simulink model "SquatTrotClimbRefined"  (R2025b)
settings: Solver=ode45  StartTime=0.0  StopTime=200  MaxStep=0.002  RelTol=0.01  AbsTol=0.01  EnableMultiTasking=on
undefined symbols (not defined in the file): a, b, c, waypoints, X, Y, Z
libraries: sm_lib x81, nesl_utility x67, hdlsllib x12, slpidlib x2, robotalgslib x1, sharedtransform x1
(part 6 of 6)

== matlab function SquatTrotClimbRefined/Rear_left_gait/MATLAB Function2 ==
  data: t input; leg_id input; q_hip output; mode_cmd input
function q_hip = hip_motion_all_legs(t, leg_id, mode_cmd)
    T_squat_start = 102;
    T_walk_start  = 130;
    
    % --- [NEW] Absolute time node for ending the walk ---
    T_walk_end    = 170;  % Start braking and retracting legs exactly at 170 seconds
    
    if (mode_cmd == 1) || (t < T_squat_start)
        q_hip = 0; return;
    end
    
    % Phase 1: Squat and stand (102s - 130s)
    if t < T_walk_start
        tau = t - T_squat_start;
        q_stand = 0; q_squat = deg2rad(35);
        T1=3; T2=15; T3=3;
        
        if tau < T1
            u = tau/T1; 
            q_hip = (1-u)*q_stand + u*q_squat;
        elseif tau < T1+T2
            q_hip = q_squat;
        elseif tau < T1+T2+T3
            u = (tau-(T1+T2))/T3; 
            q_hip = (1-u)*q_squat + u*q_stand;
        else
            q_hip = 0; 
        end
        return;
    end
    
    % Phase 2: Walking logic (130s+)
    % Relative time starting from 130s
    t_phase2 = t - T_walk_start;
    
    % ================= Tunables (Hip) =================
    ang_hip_crouch = deg2rad(30);    
    hip_swing_amp  = deg2rad(8);     
    
    ang_fwd  = ang_hip_crouch - hip_swing_amp;  
    ang_back = ang_hip_crouch + hip_swing_amp;  
    
    % ================= Timing =================
    T_crouch = 2.0;              
    T_hold   = 3.0;              
    T_ramp   = 2.0;              
    T_cycle  = 1.8;
    duty     = 0.50;             
    
    % --- [NEW] Braking and recovery time periods ---
    T_ramp_down = 2.0;    % 170s - 172s: Take 2 seconds to slowly reduce stride amplitude to 0
    T_recover   = 3.0;    % 172s - 175s: After legs stop, take 3 seconds to smoothly stand up straight (return to 0 degrees)
    
    % ================= Phase offsets =================
    phase_offset = [0.0, 0.5, 0.0, 0.5];
    phi = phase_offset(leg_id + 1);
    
    % ================= Smooth interpolators =================
    smooth = @(x) (1 - cos(x * pi)) / 2;
    
    % ==========================================================
    % Stage 1 & 2: Crouch & Hold (relative to 130s) -> (130s ~ 135s)
    % ==========================================================
    if t_phase2 < T_crouch + T_hold
        s = smooth(min(t_phase2 / T_crouch, 1.0));
        q_hip = s * ang_hip_crouch;
        return;
    end
    
    % ==========================================================
    % Stage 3: Trot & Stop (All motions after 135s)
    % ==========================================================
    t_trot = t_phase2 - T_crouch - T_hold;
    phase = mod(t_trot / T_cycle + phi, 1.0);
    
    % --- 1. Calculate theoretical pure gait trajectory (keep your already tuned normal logic) ---
    if phase < duty
        % ===== STANCE =====
        s = smooth(phase / duty);
        hip_walk  = ang_fwd + s * (ang_back - ang_fwd); 
    else
        % ===== SWING =====
        s = (phase - duty) / (1.0 - duty);
        hip_walk  = ang_back + smooth(s) * (ang_fwd - ang_back);
    end
    
    % Extract the pure stepping swing amount
    swing_offset = hip_walk - ang_hip_crouch;
    
    % --- 2. Calculate stride amplitude envelope (controls how large the step is) ---
    if t < T_walk_end
        % 135s - 170s: Start and maintain full speed
        amp_walk = smooth(min(t_trot / T_ramp, 1.0));
    elseif t < T_walk_end + T_ramp_down
        % 170s - 172s: Stride amplitude gradually decreases until stopping in place
        tau_stop = t - T_walk_end;
        amp_walk = smooth(max(1.0 - (tau_stop / T_ramp_down), 0.0));
    else
        % After 172s: Legs completely stop stepping
        amp_walk = 0.0;
    end
    
    % --- 3. Calculate base crouch angle (controls body height) ---
    if t < T_walk_end + T_ramp_down
        % Before 172s: Maintain 30 degree crouch baseline
        base_hip = ang_hip_crouch;
    elseif t < T_walk_end + T_ramp_down + T_recover
        % 172s - 175s: Smoothly stand up from 30 degree crouch back to 0 degrees
        tau_rec = t - (T_walk_end + T_ramp_down);
        s_rec = smooth(min(tau_rec / T_recover, 1.0));
        base_hip = (1.0 - s_rec) * ang_hip_crouch;
    else
        % After 175s: Completely stand straight, lock at 0 degrees, and enter wheeled driving mode
        base_hip = 0.0;
    end
    
    % --- 4. Final output = Base posture + (Stride proportion * Swing amount) ---
    q_hip = base_hip + amp_walk * swing_offset;
end

== matlab function SquatTrotClimbRefined/Rear_left_gait/MATLAB Function4 ==
  data: t input; leg_id input; q_knee output; mode_cmd input
function q_knee = knee_motion_all_legs(t, leg_id, mode_cmd)
    % --- Time Node Definitions ---
    T_squat_start = 102;
    T_walk_start  = 130; 
    
    % --- [NEW] Absolute time node for ending the walk ---
    T_walk_end    = 170;  
    
    % Phase 0: Standby
    if (mode_cmd == 1) || (t < T_squat_start)
        q_knee = 0; return;
    end
    
    % Phase 1: Squat and stand (102-130s)
    if t < T_walk_start
        tau = t - T_squat_start;
        q_stand = 0; q_squat = -deg2rad(70);
        T1=3; T2=15; T3=3;
        
        if tau < T1
            u = tau/T1; 
            q_knee = (1-u)*q_stand + u*q_squat;
        elseif tau < T1+T2
            q_knee = q_squat;
        elseif tau < T1+T2+T3
            u = (tau-(T1+T2))/T3; 
            q_knee = (1-u)*q_squat + u*q_stand;
        else
            q_knee = 0; 
        end
        return;
    end
    
    % Phase 2: Walking logic (130s+)
    % Relative time starting from 130s
    t_phase2 = t - T_walk_start;
    
    % ================= Tunables (Knee) =================
    ang_crouch = deg2rad(-40);   % Base walking crouch angle
    ang_lift   = deg2rad(-8);    % Leg lift amplitude during swing
    ang_comp   = deg2rad(-3);    % Compression amplitude during stance
    
    % ================= Timing =================
    T_crouch = 2.0;              
    T_hold   = 3.0;              
    T_ramp   = 2.0;              
    T_cycle  = 1.8;
    duty     = 0.50;             
    
    % --- [NEW] Braking and recovery time periods ---
    T_ramp_down = 2.0;    % 170s - 172s: Take 2 seconds to slowly reduce the step amplitude to 0
    T_recover   = 3.0;    % 172s - 175s: After the legs stop, take 3 seconds to smoothly stand up straight (return to 0 degrees)
    
    % ================= Phase offsets =================
    phase_offset = [0.0, 0.5, 0.0, 0.5];
    phi = phase_offset(leg_id + 1);
    
    % ================= Smooth interpolators =================
    smooth = @(x) (1 - cos(x * pi)) / 2;
    bump   = @(x) (1 - cos(2 * x * pi)) / 2;
    
    % ==========================================================
    % Stage 1 & 2: Crouch & Hold (relative to 130s) -> (130s ~ 135s)
    % ==========================================================
    if t_phase2 < T_crouch + T_hold
        s = smooth(min(t_phase2 / T_crouch, 1.0));
        q_knee = s * ang_crouch;
        return;
    end
    
    % ==========================================================
    % Stage 3: Trot & Stop (All motions after 135s)
    % ==========================================================
    t_trot = t_phase2 - T_crouch - T_hold;
    phase = mod(t_trot / T_cycle + phi, 1.0);
    
    % --- 1. Calculate theoretical pure gait trajectory (keep calculating normally to prevent phase disruption from sudden cutoff) ---
    if phase < duty
        % ===== STANCE: foot on ground =====
        knee_walk = ang_crouch + sin((phase / duty) * pi) * ang_comp;
    else
        % ===== SWING: foot in air =====
        s = (phase - duty) / (1.0 - duty);
        knee_walk = ang_crouch + bump(s) * ang_lift;
    end
    
    % Extract the pure stepping flexion/extension amount
    swing_offset = knee_walk - ang_crouch;
    
    % --- 2. Calculate stride amplitude envelope (controls how large the step is) ---
    if t < T_walk_end
        % 135s - 170s: Start and maintain full-amplitude stepping
        amp_walk = smooth(min(t_trot / T_ramp, 1.0));
    elseif t < T_walk_end + T_ramp_down
        % 170s - 172s: Stride amplitude gradually decreases until stopping in place
        tau_stop = t - T_walk_end;
        amp_walk = smooth(max(1.0 - (tau_stop / T_ramp_down), 0.0));
    else
        % After 172s: Legs completely stop stepping
        amp_walk = 0.0;
    end
    
    % --- 3. Calculate base crouch angle (controls body height) ---
    if t < T_walk_end + T_ramp_down
        % Before 172s: Maintain -40 degree crouch baseline
        base_knee = ang_crouch;
    elseif t < T_walk_end + T_ramp_down + T_recover
        % 172s - 175s: Smoothly stand up from -40 degrees back to 0 degrees
        tau_rec = t - (T_walk_end + T_ramp_down);
        s_rec = smooth(min(tau_rec / T_recover, 1.0));
        base_knee = (1.0 - s_rec) * ang_crouch;
    else
        % After 175s: Completely stand straight, lock at 0 degrees, and enter wheeled driving mode
        base_knee = 0.0;
    end
    
    % --- 4. Final synthesis ---
    % Final output = Base knee angle + (Stride proportion * Additional flexion/extension amount)
    q_knee = base_knee + amp_walk * swing_offset;
end

== matlab function SquatTrotClimbRefined/RL/MATLAB Function4 ==
  data: t input; w output
function w = wheel_speed(t)
% WHEEL_SPEED_CONTROLLER 
% This function manages the angular velocity for the rear wheels.
% Sequence: High-speed drive -> Stop -> WALKING GAIT (130s-175s) -> Low-speed drive -> Stop 10s -> Drive.

% ==========================================
% 1. Parameter Definitions (Phase 1 to 5: Initial Drive)
% ==========================================
T_start    = 105;   % Time to begin initial movement (s)
T_accel    = 2;     % Duration of linear acceleration (s)
V_max      = 100;   % Primary target velocity
V_low      = 15;    % Secondary target velocity (used in intermediate phases)
T_dec_init = 125;   % Time to start the first deceleration (s)
T_braking  = 3;     % Duration of the braking phase (s)

% ==========================================
% 2. Parameter Definitions (Phase 6+: Resume Drive after 175s)
% ==========================================
T_resume   = 175;   % Time to resume wheeled mode (Walking gait ends)
T_accel2   = 2;     % Duration to accelerate to V_low
T_hold2    = 8;     % Duration to hold V_low before the second stop
T_brake2   = 3;     % Duration of the second braking phase
T_pause2   = 2;    % Pause duration (Stop for 10s)
T_accel3   = 2;     % Final acceleration duration to V_low

% --- Pre-calculate Time Nodes for clean logic ---
T1_end_dec   = T_dec_init + T_braking; % 128s: First stop completely

T2_end_accel = T_resume + T_accel2;    % 177s: Reached 20 rad/s
T2_start_dec = T2_end_accel + T_hold2; % 185s: Start 2nd braking
T2_end_dec   = T2_start_dec + T_brake2;% 188s: Completely stopped again
T2_end_pause = T2_end_dec + T_pause2;  % 198s: 10s pause ends
T3_end_accel = T2_end_pause + T_accel3;% 200s: Final acceleration ends

% ==========================================
% 3. Logic Control and Phase Switching
% ==========================================

% --- PHASE 1: IDLE / PRE-START ---
if t < T_start
    w = 0;

% --- PHASE 2: INITIAL ACCELERATION (0 to V_max) ---
elseif t < T_start + T_accel
    u = (t - T_start) / T_accel; 
    w = u * V_max;

% --- PHASE 3: CONSTANT HIGH-SPEED CRUISE ---
elseif t < T_dec_init
    w = V_max;

% --- PHASE 4: CONTROLLED DECELERATION (V_max to 0) ---
elseif t < T1_end_dec
    u = (t - T_dec_init) / T_braking; 
    w = V_max * (1 - u);

% =========================================================
% --- PHASE 5: WALKING GAIT LOCK (128s to 175s) ---
% The robot stands still from 128s-130s, then walks from 130s-175s.
% Wheels MUST strictly remain at 0 rad/s here.
% =========================================================
elseif t < T_resume
    w = 0;

% =========================================================
% --- PHASE 6+: RESUME WHEELED MODE (175s onwards) ---
% =========================================================

% --- PHASE 6: FIRST RE-ACCELERATION (0 to V_low) ---
elseif t < T2_end_accel
    u = (t - T_resume) / T_accel2;
    w = u * V_low;

% --- PHASE 7: HOLD V_low ---
elseif t < T2_start_dec
    w = V_low;

% --- PHASE 8: SECOND DECELERATION (V_low to 0) ---
elseif t < T2_end_dec
    u = (t - T2_start_dec) / T_brake2;
    w = V_low * (1 - u);

% --- PHASE 9: THE 10-SECOND PAUSE ---
elseif t < T2_end_pause
    w = 0;

% --- PHASE 10: FINAL ACCELERATION (0 to V_low) ---
elseif t < T3_end_accel
    u = (t - T2_end_pause) / T_accel3;
    w = u * V_low;

% --- PHASE 11: CRUISE INDEFINITELY ---
else
    w = V_low;
end

end

== matlab function SquatTrotClimbRefined/RR/MATLAB Function ==
  data: mode_cmd input; alpha input; tau output; q input; dq input; q_cmd input; is_locked output; q_ref output
function [tau, is_locked, q_ref] = LockJointPD(mode_cmd, alpha, q, dq, q_cmd)
%#codegen
% mode_cmd: 0=Walk(folloew q_cmd), 1=Wheel(lock the present angle )
% alpha   : [0,1] flatten faktor(TransferFcnoutput)，0=walk, 1=leg locked
% q,dq    : joint angle/angular velocity
% q_cmd   : walking/standing angle(rad)

Kp = 1200.0;   % start value
Kd =   20.0;
tau_lim = 300.0;

m = uint8(mode_cmd ~= 0);     % uint8(0/1)
a = double(alpha);

persistent q_hold last_mode
if isempty(q_hold),    q_hold    = q;        end   % double
if isempty(last_mode), last_mode = uint8(0); end   % uint8

% step: 0->1 
if (last_mode == uint8(0)) && (m ~= uint8(0))
    q_hold = q;
end
last_mode = m;

% reference angle
q_ref  = a*q_hold + (1-a)*q_cmd;
dq_ref = 0.0;

% PD
tau = Kp*(q_ref - q) + Kd*(dq_ref - dq);

% 
tau = max(min(tau, tau_lim), -tau_lim);

% 
is_locked = (a > 0.5);     % 
end

== matlab function SquatTrotClimbRefined/FR/MATLAB Function ==
  data: mode_cmd input; alpha input; tau output; q input; dq input; q_cmd input; is_locked output; q_ref output
function [tau, is_locked, q_ref] = LockJointPD(mode_cmd, alpha, q, dq, q_cmd)
%#codegen
% mode_cmd: 0=Walk (track q_cmd), 1=Wheeled (lock current angle)
% alpha   : [0,1] smoothing factor (TransferFcn output), 0=fully walking, 1=fully locked
% q,dq    : joint angle/angular velocity
% q_cmd   : walk/stand target angle (radians)
Kp = 1200.0;   % Starting value, tune per joint
Kd =   20.0;
tau_lim = 300.0;
m = uint8(mode_cmd ~= 0);     % Standardize to uint8(0/1)
a = double(alpha);
persistent q_hold last_mode
if isempty(q_hold),    q_hold    = q;        end   % double
if isempty(last_mode), last_mode = uint8(0); end   % uint8
% Rising edge: 0->1, latch current angle
if (last_mode == uint8(0)) && (m ~= uint8(0))
    q_hold = q;
end
last_mode = m;
% Reference angle: interpolate between "hold angle" and "target angle"
q_ref  = a*q_hold + (1-a)*q_cmd;
dq_ref = 0.0;
% PD
tau = Kp*(q_ref - q) + Kd*(dq_ref - dq);
% Saturation
tau = max(min(tau, tau_lim), -tau_lim);
% Debug flag: is leg lock dominant
is_locked = (a > 0.5);     % Can also output m==1
end

== matlab function SquatTrotClimbRefined/FR/MATLAB Function1 ==
  data: mode_cmd input; alpha input; tau output; q input; dq input; q_cmd input; is_locked output; q_ref output
function [tau, is_locked, q_ref] = LockJointPD(mode_cmd, alpha, q, dq, q_cmd)
%#codegen
% mode_cmd: 0=Walk (track q_cmd), 1=Wheeled (lock current angle)
% alpha   : [0,1] smoothing factor (TransferFcn output), 0=fully walking, 1=fully locked
% q,dq    : joint angle/angular velocity
% q_cmd   : walk/stand target angle (radians)
Kp = 1200.0;   % Starting value, tune per joint
Kd =   20.0;
tau_lim = 300.0;
m = uint8(mode_cmd ~= 0);     % Standardize to uint8(0/1)
a = double(alpha);
persistent q_hold last_mode
if isempty(q_hold),    q_hold    = q;        end   % double
if isempty(last_mode), last_mode = uint8(0); end   % uint8
% Rising edge: 0->1, latch current angle
if (last_mode == uint8(0)) && (m ~= uint8(0))
    q_hold = q;
end
last_mode = m;
% Reference angle: interpolate between "hold angle" and "target angle"
q_ref  = a*q_hold + (1-a)*q_cmd;
dq_ref = 0.0;
% PD
tau = Kp*(q_ref - q) + Kd*(dq_ref - dq);
% Saturation
tau = max(min(tau, tau_lim), -tau_lim);
% Debug flag: is leg lock dominant
is_locked = (a > 0.5);     % Can also output m==1
end

== matlab function SquatTrotClimbRefined/FL/MATLAB Function ==
  data: mode_cmd input; alpha input; tau output; q input; dq input; q_cmd input; is_locked output; q_ref output
function [tau, is_locked, q_ref] = LockJointPD(mode_cmd, alpha, q, dq, q_cmd)
%#codegen
% mode_cmd: 0=Walk (track q_cmd), 1=Wheeled (lock current angle)
% alpha   : [0,1] smoothing factor (TransferFcn output), 0=fully walking, 1=fully locked
% q,dq    : joint angle/angular velocity
% q_cmd   : walk/stand target angle (radians)
Kp = 1200.0;   % Starting value, tune per joint
Kd =   20.0;
tau_lim = 300.0;
m = uint8(mode_cmd ~= 0);     % Standardize to uint8(0/1)
a = double(alpha);
persistent q_hold last_mode
if isempty(q_hold),    q_hold    = q;        end   % double
if isempty(last_mode), last_mode = uint8(0); end   % uint8
% Rising edge: 0->1, latch current angle
if (last_mode == uint8(0)) && (m ~= uint8(0))
    q_hold = q;
end
last_mode = m;
% Reference angle: interpolate between "hold angle" and "target angle"
q_ref  = a*q_hold + (1-a)*q_cmd;
dq_ref = 0.0;
% PD
tau = Kp*(q_ref - q) + Kd*(dq_ref - dq);
% Saturation
tau = max(min(tau, tau_lim), -tau_lim);
% Debug flag: is leg lock dominant
is_locked = (a > 0.5);     % Can also output m==1
end

== matlab function SquatTrotClimbRefined/FL/MATLAB Function1 ==
  data: mode_cmd input; alpha input; tau output; q input; dq input; q_cmd input; is_locked output; q_ref output
function [tau, is_locked, q_ref] = LockJointPD(mode_cmd, alpha, q, dq, q_cmd)
%#codegen
% mode_cmd: 0=Walk (track q_cmd), 1=Wheeled (lock current angle)
% alpha   : [0,1] smoothing factor (TransferFcn output), 0=fully walking, 1=fully locked
% q,dq    : joint angle/angular velocity
% q_cmd   : walk/stand target angle (radians)
Kp = 1200.0;   % Starting value, tune per joint
Kd =   20.0;
tau_lim = 300.0;
m = uint8(mode_cmd ~= 0);     % Standardize to uint8(0/1)
a = double(alpha);
persistent q_hold last_mode
if isempty(q_hold),    q_hold    = q;        end   % double
if isempty(last_mode), last_mode = uint8(0); end   % uint8
% Rising edge: 0->1, latch current angle
if (last_mode == uint8(0)) && (m ~= uint8(0))
    q_hold = q;
end
last_mode = m;
% Reference angle: interpolate between "hold angle" and "target angle"
q_ref  = a*q_hold + (1-a)*q_cmd;
dq_ref = 0.0;
% PD
tau = Kp*(q_ref - q) + Kd*(dq_ref - dq);
% Saturation
tau = max(min(tau, tau_lim), -tau_lim);
% Debug flag: is leg lock dominant
is_locked = (a > 0.5);     % Can also output m==1
end

== matlab function SquatTrotClimbRefined/RL/MATLAB Function ==
  data: mode_cmd input; alpha input; tau output; q input; dq input; q_cmd input; is_locked output; q_ref output
function [tau, is_locked, q_ref] = LockJointPD(mode_cmd, alpha, q, dq, q_cmd)
%#codegen
% mode_cmd: 0=Walk (track q_cmd), 1=Wheeled (lock current angle)
% alpha   : [0,1] smoothing factor (TransferFcn output), 0=fully walking, 1=fully locked
% q,dq    : joint angle/angular velocity
% q_cmd   : walk/stand target angle (radians)
Kp = 1200.0;   % Starting value, tune per joint
Kd =   20.0;
tau_lim = 300.0;
m = uint8(mode_cmd ~= 0);     % Standardize to uint8(0/1)
a = double(alpha);
persistent q_hold last_mode
if isempty(q_hold),    q_hold    = q;        end   % double
if isempty(last_mode), last_mode = uint8(0); end   % uint8
% Rising edge: 0->1, latch current angle
if (last_mode == uint8(0)) && (m ~= uint8(0))
    q_hold = q;
end
last_mode = m;
% Reference angle: interpolate between "hold angle" and "target angle"
q_ref  = a*q_hold + (1-a)*q_cmd;
dq_ref = 0.0;
% PD
tau = Kp*(q_ref - q) + Kd*(dq_ref - dq);
% Saturation
tau = max(min(tau, tau_lim), -tau_lim);
% Debug flag: is leg lock dominant
is_locked = (a > 0.5);     % Can also output m==1
end
